simulink model "simulaciones simulink"  (R2016a)
settings: Solver=VariableStepAuto  StartTime=0.0  StopTime=0.01  RelTol=1e-3
values from neighbouring files (symbols this model uses):
  a = 1    [simulaciones matlab.m]
  den = [(r1*r3*c1*c2) (r1*r3*c2)*((1/r1)+(1/r2)+(1/r3)) (r1/r2)]    [simulaciones matlab.m]
  f = 500    [simulaciones matlab.m]
  fn = 500    [simulaciones matlab.m]
  Fs = 10*f    (= 5000)    [simulaciones matlab.m]
  num = -1    [simulaciones matlab.m]
  Ts = 1/(10*fn)    (= 0.0002)    [simulaciones matlab.m]
undefined symbols (not defined in the file or in its folder): denz, numz
settings Model: Creator=sebas  LastModifiedBy=sebas

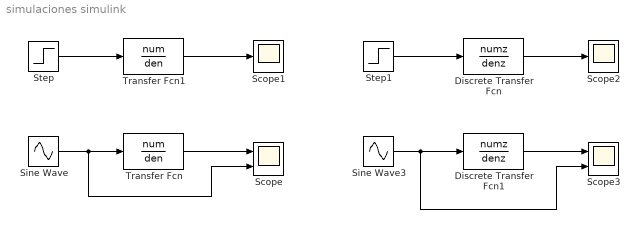
== system simulaciones simulink ==
  Discrete Transfer Fcn : DiscreteTransferFcn  Numerator=numz  Denominator=denz  SampleTime=0.0001
  Discrete Transfer Fcn1 : DiscreteTransferFcn  Numerator=numz  Denominator=denz  SampleTime=0.0001
  Scope : Scope  NumInputPorts=2
  Scope1 : Scope
  Scope2 : Scope
  Scope3 : Scope  NumInputPorts=2
  Sine Wave : Sin  Amplitude=a  Frequency=f  SampleTime=1/(Fs*100)
  Sine Wave3 : Sin  Amplitude=a  Frequency=fn  SampleTime=Ts
  Step : Step  Time=0  SampleTime=0
  Step1 : Step  Time=0  SampleTime=0
  Transfer Fcn : TransferFcn  Numerator=num  Denominator=den
  Transfer Fcn1 : TransferFcn  Numerator=num  Denominator=den
  wires:
  Step/1 -> Transfer Fcn1/1
  Transfer Fcn1/1 -> Scope1/1
  Transfer Fcn/1 -> Scope/1
  Sine Wave/1 -> Scope/2, Transfer Fcn/1
  Sine Wave3/1 -> Scope3/2, Discrete Transfer Fcn1/1
  Discrete Transfer Fcn1/1 -> Scope3/1
  Step1/1 -> Discrete Transfer Fcn/1
  Discrete Transfer Fcn/1 -> Scope2/1
